simulink model "dynamic"  (R2023b)
settings: Solver=VariableStepAuto  StartTime=0.0  StopTime=5  MaxStep=1e-5  RelTol=1e-3
values from neighbouring files (symbols this model uses):
  phi0 = 0    [main.m]
  phidot0 = 0    [main.m]
  psif0 = 0    [main.m]
  psifdot0 = 0    [main.m]
  psir0 = 0    [main.m]
  psirdot0 = 0    [main.m]
  rho0 = 0    [main.m]
  rhodot0 = 0    [main.m]
  theta_dot_fl0 = xdot0*cos(car.toe.fl*pi/180)/car.tr.fl    [main.m]
  theta_dot_fr0 = xdot0*cos(car.toe.fr*pi/180)/car.tr.fr    [main.m]
  theta_dot_rl0 = xdot0*cos(car.toe.rl*pi/180)/car.tr.rl    [main.m]
  theta_dot_rr0 = xdot0*cos(car.toe.rr*pi/180)/car.tr.rr    [main.m]
  x0 = 0    [main.m]
  xdot0 = 10    [main.m]
  y0 = 0    [main.m]
  ydot0 = 0    [main.m]
  Zs0 = 0    [main.m]
  Zsdot0 = 0    [main.m]
  Zufl0 = 0    [main.m]
  Zufldot0 = 0    [main.m]
  Zufr0 = 0    [main.m]
  Zufrdot0 = 0    [main.m]
  Zurl0 = 0    [main.m]
  Zurldot0 = 0    [main.m]
  Zurr0 = 0    [main.m]
  Zurrdot0 = 0    [main.m]
undefined symbols (not defined in the file or in its folder): car
libraries: simulink x4, spsFirstOrderFilterLib x1
(part 1 of 2)
settings Model: Creator=Admin  LastModifiedBy=nathan

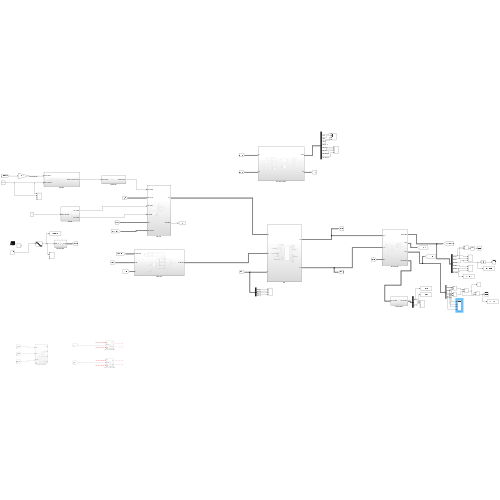
[thumbnail: Simulink's stored preview of the top-level diagram]
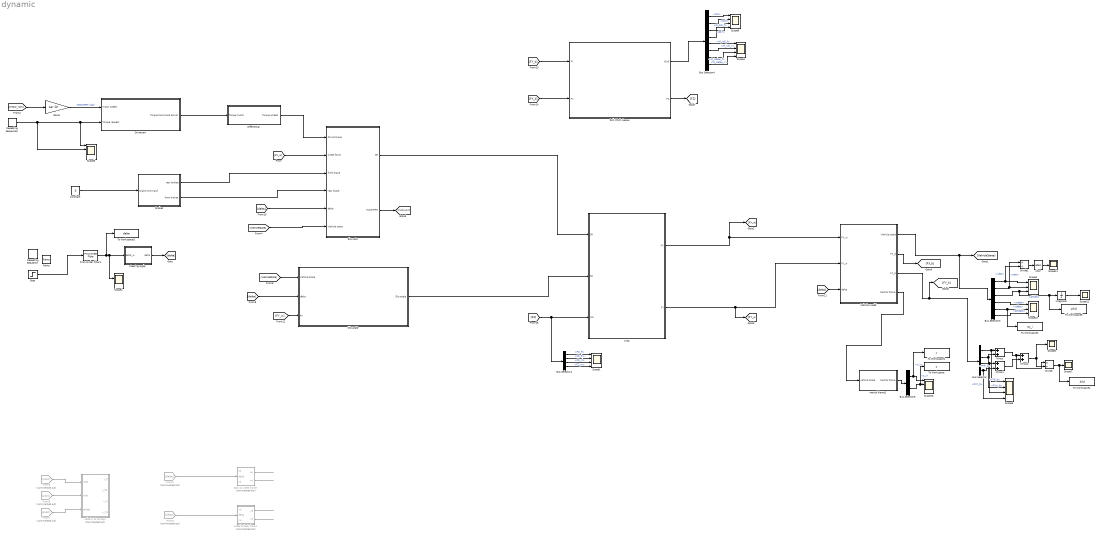
== system dynamic ==
  Atan : Trigonometry  Operator=atan
  Brakes : Subsystem
  Bus Selector : BusSelector  OutputSignals=FYfr_b,FYfl_b,FYrr_b,FYrl_b
  Bus Selector1 : BusSelector  OutputSignals=FZ_fl,FZ_fr,FZ_rl,FZ_rr
  Bus Selector3 : BusSelector  OutputSignals=xdot,ydot,phidot,xddot,yddot,phiddot
  Bus Selector4 : BusSelector  OutputSignals=cts,psif.psif,psir.psir,M_arb.M_arb_f,Roll moment.M_roll_f,Roll moment.M_roll_r,Roll moment.M_inelas_f,Roll moment.M_inelas_r
  Bus Selector5 : BusSelector  OutputSignals=x_i,y_i
  Constant : Constant  Value=0
  Differential : Subsystem
  Divide : Product  Inputs=*/
  Divide1 : Product  Inputs=*/
  Drivetrain : Subsystem
  First-Order Filter1 : spsFirstOrderFilterLib/First-Order Filter  FilterType=Lowpass  Tc=0  Ts=0  Initialize=on  Vac_Init=[0, 0, 60]  Vdc_Init=0  PlotResponse=off  FreqRange="[0,  200,  1]"
  From1 : From  Commented=on  GotoTag=delta
  From3 : From  Commented=on  GotoTag=delta
  From5 : From  Commented=on  GotoTag=xdot
  From6 : From  Commented=on  GotoTag=ydot
  From7 : From  Commented=on  GotoTag=phidot
  Gain5 : Gain  Gain=car.Gr
  Inertial frame2 : Subsystem
  Integrator : Integrator
  Minus : Sum
  Minus1 : Sum
  Minus2 : Sum
  Ramp : simulink/Sources/Ramp  slope=1  start=1  InitialOutput=0
  Repeating Sequence : simulink/Sources/Repeating Sequence  rep_seq_t=[0 1 1.1 10]  rep_seq_y=[0 0 10 25]
  Repeating Sequence2 : simulink/Sources/Repeating Sequence  rep_seq_t=[0 0.05 1 1.05 2 2.05 20]  rep_seq_y=[0 0 0 0 0 0 0]
  "Roll, Pitch, Heave" : Subsystem
  Scope{1,3..6,9,13} (7 alike) : Scope  NumInputPorts=4
  Scope10 : Scope  NumInputPorts=3
  Scope{7..8,11..12} (4 alike) : Scope
  Scope2 : Scope  NumInputPorts=3
  Slip angle : Subsystem
  Slip ratio : Subsystem
  Step : Step  After=10  SampleTime=0
  To Workspace : ToWorkspace  VariableName=y  SampleTime=-1
  To Workspace1 : ToWorkspace  VariableName=x  SampleTime=-1
  To Workspace2 : ToWorkspace  VariableName=ay_i  SampleTime=-1
  To Workspace3 : ToWorkspace  VariableName=delta  SampleTime=-1
  To Workspace4 : ToWorkspace  VariableName=AYd  SaveFormat=Timeseries  SampleTime=-1
  To Workspace5 : ToWorkspace  VariableName=phid  SaveFormat=Timeseries  SampleTime=-1
  Vehicle model : Subsystem
  body to wheel frame : Subsystem  Commented=on
  steering angle : Subsystem
  tires : Subsystem
  velocity at corners : Subsystem  Commented=on
  wheel to body frame : Subsystem  Commented=on
  wires:
  [motor_rpm] -> Gain5/1
  Gain5/1 -> Drivetrain/1(motor speed)  "MotorRPM (rad)"
  Constant/1 -> Brakes/1(brake command)
  ? -> body to wheel frame/1(xb)
  From1/1 -> body to wheel frame/2(delta)
  ? -> body to wheel frame/3(yb)
  body to wheel frame/1(xw) -> ?
  body to wheel frame/2(yw) -> ?
  wheel to body frame/2(yb) -> ?
  wheel to body frame/1(xb) -> ?
  ? -> wheel to body frame/3(yw)
  From3/1 -> wheel to body frame/2(delta)
  ? -> wheel to body frame/1(xw)
  From5/1 -> velocity at corners/1(xdot)
  From6/1 -> velocity at corners/2(ydot)
  From7/1 -> velocity at corners/3(phidot)
  [FX_w] -> Slip ratio/2(wheel force)
  Brakes/1(rear brakes) -> Slip ratio/3(front brake)
  Brakes/2(front brakes) -> Slip ratio/4(rear brake)
  steering angle/1(delta) -> [delta]
  [delta] -> Slip ratio/5(delta)
  [delta] -> Vehicle model/3(delta)
  Vehicle model/1(Vehicle state) -> Bus Selector3/1, [VehicleState]
  [VehicleState] -> Slip ratio/6(Vehicle state)
  [VehicleState] -> Slip angle/1(Vehicle state)
  [delta] -> Slip angle/2(delta)
  [FY_w] -> Slip angle/3(FY)
  Vehicle model/4(Inertial frame) -> Inertial frame2/1(vehicle state)
  Slip ratio/2(MotorRPM) -> [motor_rpm]
  Drivetrain/1(Torque Command actual) -> Differential/1(Torque motor)
  Differential/1(Torque wheels) -> Slip ratio/1(Drive torque)
  [FX_b] -> "Roll, Pitch, Heave"/2(FX)
  Vehicle model/2(FX_b) -> [FX_b]
  Vehicle model/3(FY_b) -> Bus Selector/1, [FY_b]
  "Roll, Pitch, Heave"/1(BUS) -> Bus Selector4/1
  "Roll, Pitch, Heave"/2(FZ) -> [FZ]
  tires/2(FY) -> Vehicle model/2(FY_w), [FY_w]
  tires/1(FX) -> [FX_w], Vehicle model/1(FX_w)
  Slip ratio/1(SR) -> tires/1(SR)
  Slip angle/1(Slip angle) -> tires/2(SA)
  [FZ] -> Bus Selector1/1, tires/3(In3)
  Bus Selector1/1 -> Scope1/1  "<FZ_fl>"
  Bus Selector1/2 -> Scope1/2  "<FZ_fr>"
  Bus Selector1/3 -> Scope1/3  "<FZ_rl>"
  Bus Selector1/4 -> Scope1/4  "<FZ_rr>"
  Bus Selector4/5 -> Scope3/1  "<M_roll_f>"
  Bus Selector4/6 -> Scope3/2  "<M_roll_r>"
  Bus Selector4/7 -> Scope3/3  "<M_inelas_f>"
  Bus Selector4/8 -> Scope3/4  "<M_inelas_r>"
  Bus Selector4/1 -> Scope6/1  "<cts>"
  Bus Selector4/2 -> Scope6/2  "<psif>"
  Bus Selector4/3 -> Scope6/3  "<psir>"
  Bus Selector4/4 -> Scope6/4  "<M_arb_f>"
  [FY_b] -> "Roll, Pitch, Heave"/1(FY)
  Repeating Sequence2/1 -> Scope5/1, Drivetrain/2(Torque request), Scope5/2
  Bus Selector3/1 -> Divide1/2, Scope2/1  "<xdot>"
  Bus Selector3/2 -> Divide1/1, Scope2/2  "<ydot>"
  Bus Selector3/3 -> To Workspace5/1, Integrator/1, Scope2/3  "<phidot>"
  Bus Selector/1 -> Scope9/1, Minus/1  "<FYfr_b>"
  Bus Selector/2 -> Minus/2, Scope9/2  "<FYfl_b>"
  Bus Selector/3 -> Scope9/3, Minus1/1  "<FYrr_b>"
  Bus Selector/4 -> Scope9/4, Minus1/2  "<FYrl_b>"
  Minus/1 -> Divide/1, Minus2/1
  Minus1/1 -> Minus2/2
  Divide/1 -> To Workspace4/1, Scope7/1
  Minus2/1 -> Scope8/1, Divide/2
  First-Order Filter1/1 -> To Workspace3/1, Scope4/2, steering angle/1(delta_w)
  Bus Selector3/4 -> Scope10/1  "<xddot>"
  Bus Selector3/5 -> Scope10/2, To Workspace2/1  "<yddot>"
  Bus Selector3/6 -> Scope10/3  "<phiddot>"
  Divide1/1 -> Atan/1
  Atan/1 -> Scope11/1
  Integrator/1 -> Scope12/1
  Inertial frame2/1(inertial frame) -> Bus Selector5/1
  Bus Selector5/1 -> To Workspace1/1, Scope13/1  "<x_i>"
  Bus Selector5/2 -> To Workspace/1, Scope13/2  "<y_i>"
  Step/1 -> First-Order Filter1/1

== system dynamic/Brakes ==
  brake command : Inport
  Gain12 : Gain  Gain=9.81*car.m
  Gain13 : Gain  Gain=car.brakebias
  Gain14 : Gain  Gain=0.5*car.tr.fr
  Gain9 : Gain  Gain=0.5*car.tr.rr
  Minus4 : Sum  Inputs=+-
  rear brakes : Outport
  front brakes : Outport  Port=2
  wires:
  Gain9/1 -> front brakes/1  "front brake"
  brake command/1 -> Gain12/1
  Gain13/1 -> Gain9/1, Minus4/2
  Gain12/1 -> Minus4/1, Gain13/1
  Minus4/1 -> Gain14/1  "rear brake torque total"
  Gain14/1 -> rear brakes/1  "rear brake"

== system dynamic/Differential ==
  Torque motor : Inport
  Gain : Gain  Gain=0.5
  Torque wheels : Outport
  wires:
  Torque motor/1 -> Gain/1
  Gain/1 -> Torque wheels/1

== system dynamic/Drivetrain ==
  motor speed : Inport
  Torque request : Inport  Port=2
  1-D Lookup Table : Lookup_n-D  NumberOfTableDimensions=1  BreakpointsForDimension1=car.motor(1,:)  Table=car.motor(2,:)  InternalRulePriority=Speed  RndMeth=Simplest
  Constant : Constant  Value=0
  Constant3 : Constant  Value=0
  Gain6 : Gain  Gain=30/pi
  Product : Product
  Saturation Dynamic : simulink/Discontinuities/Saturation Dynamic  OutMin=[]  OutMax=[]  OutDataTypeStr=Inherit: Same as second input  OutDataType=fixdt(1, 16)  OutScaling=2^-10  DoSatur=off
  Scope1 : Scope
  Scope2 : Scope
  Scope5 : Scope
  Switch : Switch  Criteria=u2 > Threshold  Threshold=7000  SaturateOnIntegerOverflow=off  InputSameDT=off
  gear ratio : Gain  Gain=car.Gr
  Torque Command actual : Outport
  wires:
  Constant3/1 -> Switch/1
  1-D Lookup Table/1 -> Saturation Dynamic/1
  Gain6/1 -> Scope2/1, Switch/2, 1-D Lookup Table/1  "MotorRPM (RPM)"
  motor speed/1 -> Product/1, Gain6/1, Product/2  "MotorRPM (rad)"
  Saturation Dynamic/1 -> Switch/3  "Torque command"
  Switch/1 -> Scope1/1, gear ratio/1  "Torque Command actual"
  Product/1 -> Scope5/1
  Constant/1 -> Saturation Dynamic/3
  Torque request/1 -> Saturation Dynamic/2
  gear ratio/1 -> Torque Command actual/1

== system dynamic/Inertial frame2 ==
  vehicle state : Inport
  Bus Creator2 : BusCreator  Inputs=3
  Bus Selector2 : BusSelector  OutputSignals=xdddot_if,yddot_if,phi
  Cos : Trigonometry  Operator=cos
  Cos1 : Trigonometry
  Integrator1 : Integrator  InitialCondition=ydot0
  Integrator2 : Integrator  InitialCondition=xdot0
  Integrator3 : Integrator  InitialCondition=x0
  Integrator4 : Integrator  InitialCondition=y0
  Minus : Sum  Inputs=+-
  Minus1 : Sum
  Product{,1..3} (4 alike) : Product
  inertial frame : Outport
  wires:
  Integrator1/1 -> Integrator4/1  "ydot_i"
  Bus Selector2/3 -> Cos/1, Bus Creator2/3, Cos1/1  "<phi>"
  Cos1/1 -> Product1/2, Product2/2
  Bus Creator2/1 -> inertial frame/1
  Bus Selector2/2 -> Product3/1, Product1/1  "<yddot_if>"
  Cos/1 -> Product/2, Product3/2
  Product3/1 -> Minus1/2
  Product2/1 -> Minus1/1
  Bus Selector2/1 -> Product2/1, Product/1  "<xdddot_if>"
  Integrator2/1 -> Integrator3/1  "xdot_i"
  Minus1/1 -> Integrator1/1  "yydot_i"
  Minus/1 -> Integrator2/1  "xdot_i"
  Product/1 -> Minus/1
  Product1/1 -> Minus/2
  vehicle state/1 -> Bus Selector2/1
  Integrator3/1 -> Bus Creator2/1  "x_i"
  Integrator4/1 -> Bus Creator2/2  "y_i"

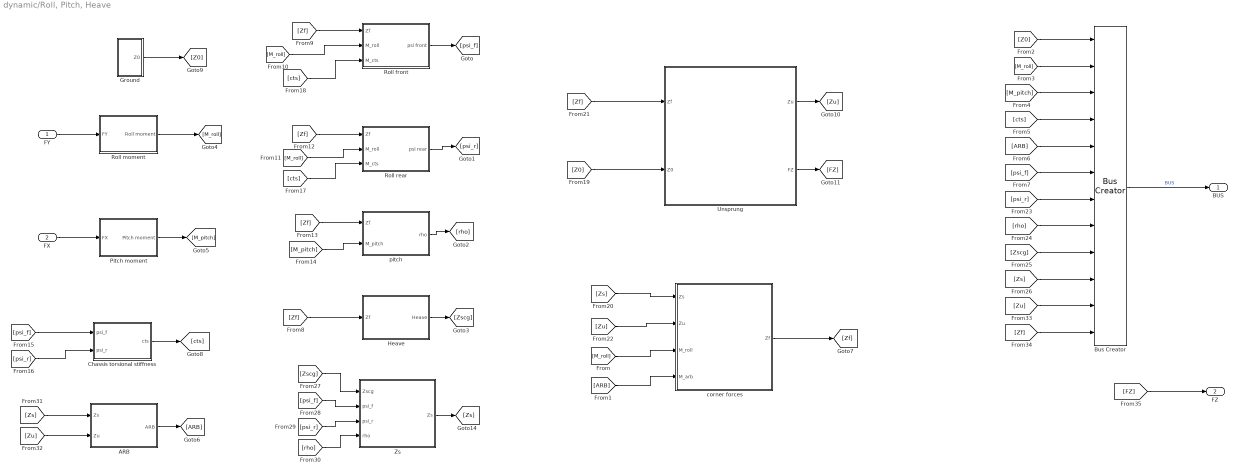
== system dynamic/Roll, Pitch, Heave ==
  FY : Inport
  FX : Inport  Port=2
  ARB : Subsystem
  Bus Creator : BusCreator  Inputs=12
  Chassis torsional stiffness : Subsystem
  Ground : Subsystem
  Heave : Subsystem
  Pitch moment : Subsystem
  Roll front : Subsystem
  Roll moment : Subsystem
  Roll rear : Subsystem
  Unsprung : Subsystem
  Zs : Subsystem
  corner forces : Subsystem
  pitch : Subsystem
  BUS : Outport
  FZ : Outport  Port=2
  wires:
  FY/1 -> Roll moment/1(FY)
  FX/1 -> Pitch moment/1(FX)
  Roll front/1(psi front) -> [psi_f]
  Roll rear/1(psi rear) -> [psi_r]
  pitch/1(rho) -> [rho]
  Heave/1(Heave) -> [Zscg]
  Roll moment/1(Roll moment) -> [M_roll]
  Pitch moment/1(Pitch moment) -> [M_pitch]
  ARB/1(ARB) -> [ARB]
  [Zf] -> Heave/1(Zf)
  [Zf] -> Roll front/1(Zf)
  [M_roll] -> Roll front/2(M_roll)
  [M_roll] -> Roll rear/2(M_roll)
  [Zf] -> Roll rear/1(Zf)
  [Zf] -> pitch/1(Zf)
  [M_pitch] -> pitch/2(M_pitch)
  Chassis torsional stiffness/1(cts) -> [cts]
  [psi_f] -> Chassis torsional stiffness/1(psi_f)
  [psi_r] -> Chassis torsional stiffness/2(psi_r)
  [cts] -> Roll front/3(M_cts)
  [cts] -> Roll rear/3(M_cts)
  Ground/1(Z0) -> [Z0]
  [Zscg] -> Zs/1(Zscg)
  [psi_f] -> Zs/2(psi_f)
  [psi_r] -> Zs/3(psi_r)
  [rho] -> Zs/4(rho)
  Zs/1(Zs) -> [Zs]
  [Zs] -> ARB/1(Zs)
  [Zf] -> Unsprung/1(Zf)
  [Z0] -> Unsprung/2(Z0)
  Unsprung/1(Zu) -> [Zu]
  [Zu] -> ARB/2(Zu)
  [Zs] -> corner forces/1(Zs)
  [Zu] -> corner forces/2(Zu)
  [M_roll] -> corner forces/3(M_roll)
  [ARB] -> corner forces/4(M_arb)
  corner forces/1(Zf) -> [Zf]
  [Z0] -> Bus Creator/1
  [M_roll] -> Bus Creator/2
  [M_pitch] -> Bus Creator/3
  [cts] -> Bus Creator/4
  [ARB] -> Bus Creator/5
  [psi_f] -> Bus Creator/6
  [psi_r] -> Bus Creator/7
  [rho] -> Bus Creator/8
  [Zscg] -> Bus Creator/9
  [Zs] -> Bus Creator/10
  [Zu] -> Bus Creator/11
  [Zf] -> Bus Creator/12
  Bus Creator/1 -> BUS/1  "BUS"
  Unsprung/2(FZ) -> [FZ]
  [FZ] -> FZ/1

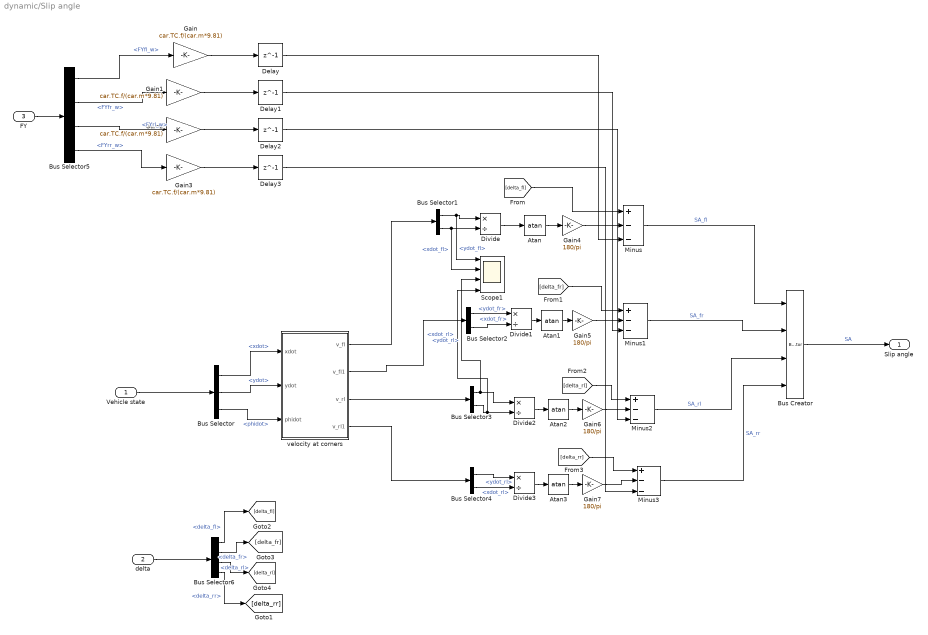
== system dynamic/Slip angle ==
  Vehicle state : Inport
  delta : Inport  Port=2
  FY : Inport  Port=3
  Atan{,1..3} (4 alike) : Trigonometry  Operator=atan
  Bus Creator : BusCreator  Inputs=4
  Bus Selector : BusSelector  OutputSignals=xdot,ydot,phidot
  Bus Selector1 : BusSelector  OutputSignals=ydot_fl,xdot_fl
  Bus Selector2 : BusSelector  OutputSignals=ydot_fr,xdot_fr
  Bus Selector3 : BusSelector  OutputSignals=ydot_rl,xdot_rl
  Bus Selector4 : BusSelector  OutputSignals=ydot_rl,xdot_rl
  Bus Selector5 : BusSelector  OutputSignals=FYfl_w,FYfr_w,FYrl_w,FYrr_w
  Bus Selector6 : BusSelector  OutputSignals=delta_fl,delta_fr,delta_rl,delta_rr
  Delay{,1..3} (4 alike) : Delay  DelayLength=1
  Divide{,1..3} (4 alike) : Product  Inputs=*/
  Gain{,1..3} (4 alike) : Gain  Gain=car.TC.f/(car.m*9.81)
  Gain{4..7} (4 alike) : Gain  Gain=180/pi
  Minus{,1..3} (4 alike) : Sum  Inputs=+--
  Scope1 : Scope  NumInputPorts=4
  velocity at corners : Subsystem
  Slip angle : Outport
  wires:
  Vehicle state/1 -> Bus Selector/1
  Bus Selector/1 -> velocity at corners/1(xdot)  "<xdot>"
  Bus Selector/2 -> velocity at corners/2(ydot)  "<ydot>"
  Bus Selector/3 -> velocity at corners/3(phidot)  "<phidot>"
  velocity at corners/1(v_fl) -> Bus Selector1/1
  Bus Selector1/1 -> Scope1/1, Divide/1  "<ydot_fl>"
  Bus Selector1/2 -> Scope1/2, Divide/2  "<xdot_fl>"
  Divide/1 -> Atan/1
  Divide1/1 -> Atan1/1
  velocity at corners/2(v_fl1) -> Bus Selector2/1
  Divide2/1 -> Atan2/1
  Divide3/1 -> Atan3/1
  velocity at corners/3(v_rl) -> Bus Selector3/1
  velocity at corners/4(v_rl1) -> Bus Selector4/1
  Bus Selector4/1 -> Divide3/1  "<ydot_rl>"
  Bus Selector4/2 -> Divide3/2  "<xdot_rl>"
  Bus Selector3/1 -> Scope1/3, Divide2/1  "<ydot_rl>"
  Bus Selector3/2 -> Divide2/2, Scope1/4  "<xdot_rl>"
  Bus Selector2/1 -> Divide1/1  "<ydot_fr>"
  Bus Selector2/2 -> Divide1/2  "<xdot_fr>"
  Atan/1 -> Gain4/1
  Bus Selector6/2 -> [delta_fr]  "<delta_fr>"
  Bus Selector6/4 -> [delta_rr]  "<delta_rr>"
  Bus Selector6/3 -> [delta_rl]  "<delta_rl>"
  Bus Selector6/1 -> [delta_fl]  "<delta_fl>"
  delta/1 -> Bus Selector6/1
  [delta_fl] -> Minus/1
  Atan1/1 -> Gain5/1
  [delta_fr] -> Minus1/1
  Atan3/1 -> Gain7/1
  Atan2/1 -> Gain6/1
  [delta_rl] -> Minus2/1
  [delta_rr] -> Minus3/1
  FY/1 -> Bus Selector5/1
  Bus Selector5/1 -> Gain/1  "<FYfl_w>"
  Bus Selector5/2 -> Gain1/1  "<FYfr_w>"
  Bus Selector5/3 -> Gain2/1  "<FYrl_w>"
  Bus Selector5/4 -> Gain3/1  "<FYrr_w>"
  Gain/1 -> Delay/1
  Gain1/1 -> Delay1/1
  Gain2/1 -> Delay2/1
  Gain3/1 -> Delay3/1
  Minus/1 -> Bus Creator/1  "SA_fl"
  Minus1/1 -> Bus Creator/2  "SA_fr"
  Minus2/1 -> Bus Creator/3  "SA_rl"
  Minus3/1 -> Bus Creator/4  "SA_rr"
  Bus Creator/1 -> Slip angle/1  "SA"
  Delay/1 -> Minus/3
  Delay1/1 -> Minus1/3
  Delay2/1 -> Minus2/3
  Delay3/1 -> Minus3/3
  Gain4/1 -> Minus/2
  Gain5/1 -> Minus1/2
  Gain6/1 -> Minus2/2
  Gain7/1 -> Minus3/2

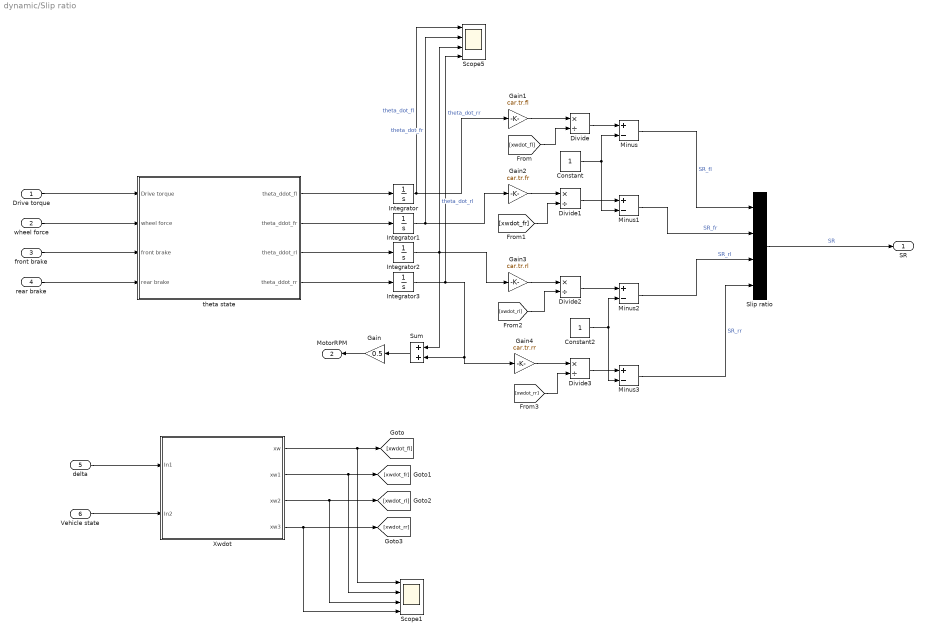
== system dynamic/Slip ratio ==
  Drive torque : Inport
  wheel force : Inport  Port=2
  front brake : Inport  Port=3
  rear brake : Inport  Port=4
  delta : Inport  Port=5
  Vehicle state : Inport  Port=6
  Constant : Constant
  Constant2 : Constant
  Divide{,1..3} (4 alike) : Product  Inputs=*/
  Gain : Gain  Gain=0.5
  Gain1 : Gain  Gain=car.tr.fl
  Gain2 : Gain  Gain=car.tr.fr
  Gain3 : Gain  Gain=car.tr.rl
  Gain4 : Gain  Gain=car.tr.rr
  Integrator : Integrator  InitialCondition=theta_dot_fr0
  Integrator1 : Integrator  InitialCondition=theta_dot_fl0
  Integrator2 : Integrator  InitialCondition=theta_dot_rl0
  Integrator3 : Integrator  InitialCondition=theta_dot_rr0
  Minus{,1..3} (4 alike) : Sum  Inputs=+-
  Scope1 : Scope  NumInputPorts=4
  Scope5 : Scope  NumInputPorts=4
  Slip ratio : BusCreator  Inputs=4
  Sum : Sum
  Xwdot : Subsystem
  theta state : Subsystem
  SR : Outport
  MotorRPM : Outport  Port=2
  wires:
  Integrator3/1 -> Scope5/4, Sum/2, Gain4/1  "theta_dot_rr"
  Integrator/1 -> Scope5/1, Gain1/1  "theta_dot_fl"
  Integrator2/1 -> Scope5/3, Sum/1, Gain3/1  "theta_dot_rl"
  theta state/3(theta_ddot_rl) -> Integrator2/1
  theta state/4(theta_ddot_rr) -> Integrator3/1
  theta state/2(theta_ddot_fr) -> Integrator1/1
  Integrator1/1 -> Scope5/2, Gain2/1  "theta_dot_fr"
  theta state/1(theta_ddot_fl) -> Integrator/1
  wheel force/1 -> theta state/2(wheel force)
  Gain2/1 -> Divide1/1
  Drive torque/1 -> theta state/1(Drive torque)
  Gain3/1 -> Divide2/1
  front brake/1 -> theta state/3(front brake)
  rear brake/1 -> theta state/4(rear brake)
  Gain1/1 -> Divide/1
  [xwdot_fl] -> Divide/2
  [xwdot_fr] -> Divide1/2
  [xwdot_rl] -> Divide2/2
  [xwdot_rr] -> Divide3/2
  Gain4/1 -> Divide3/1
  Divide/1 -> Minus/1
  Constant/1 -> Minus/2, Minus1/2
  Divide1/1 -> Minus1/1
  Divide2/1 -> Minus2/1
  Divide3/1 -> Minus3/1
  Constant2/1 -> Minus2/2, Minus3/2
  Minus/1 -> Slip ratio/1  "SR_fl"
  Minus1/1 -> Slip ratio/2  "SR_fr"
  Minus2/1 -> Slip ratio/3  "SR_rl"
  Minus3/1 -> Slip ratio/4  "SR_rr"
  Slip ratio/1 -> SR/1  "SR"
  delta/1 -> Xwdot/1(In1)
  Vehicle state/1 -> Xwdot/2(In2)
  Xwdot/2(xw1) -> Scope1/2, [xwdot_fr]
  Xwdot/3(xw2) -> Scope1/3, [xwdot_rl]
  Xwdot/4(xw3) -> Scope1/4, [xwdot_rr]
  Sum/1 -> Gain/1
  Gain/1 -> MotorRPM/1
  Xwdot/1(xw) -> Scope1/1, [xwdot_fl]

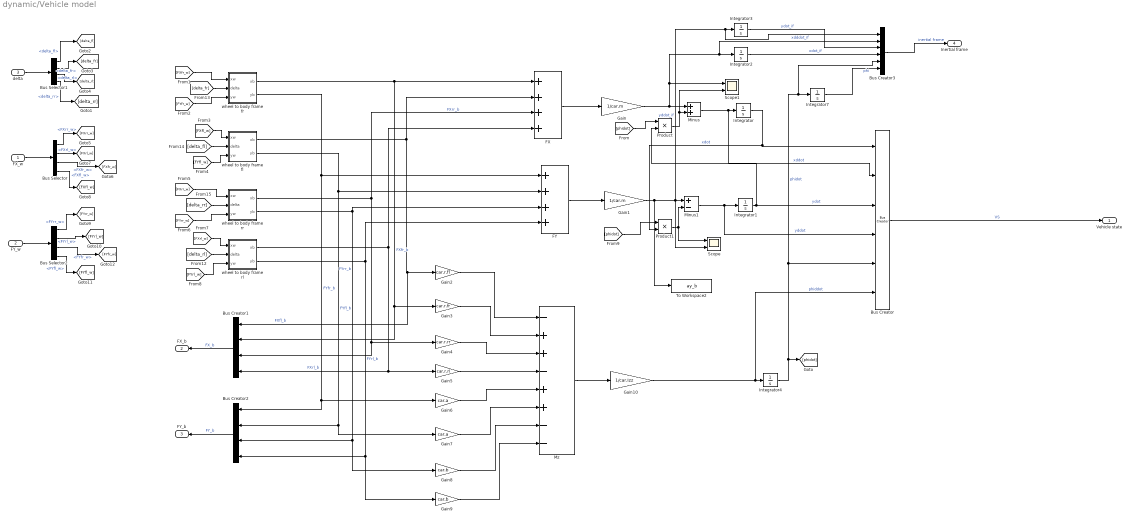
== system dynamic/Vehicle model ==
  FX_w : Inport
  FY_w : Inport  Port=2
  delta : Inport  Port=3
  Bus Creator : BusCreator  Inputs=6
  Bus Creator1 : BusCreator  Inputs=4
  Bus Creator2 : BusCreator  Inputs=4
  Bus Creator3 : BusCreator  Inputs=6
  Bus Selector : BusSelector  OutputSignals=FXrr_w,FXrl_w,FXfr_w,FXfl_w
  Bus Selector1 : BusSelector  OutputSignals=delta_fl,delta_fr,delta_rl,delta_rr
  Bus Selector2 : BusSelector  OutputSignals=FYrr_w,FYrl_w,FYfr_w,FYfl_w
  FX : Sum  Inputs=++++
  FY : Sum  Inputs=++++
  Gain : Gain  Gain=1/car.m
  Gain1 : Gain  Gain=1/car.m
  Gain10 : Gain  Gain=1/car.Izz
  Gain2 : Gain  Gain=car.r.fl
  Gain3 : Gain  Gain=car.r.fr
  Gain4 : Gain  Gain=car.r.rr
  Gain5 : Gain  Gain=car.r.rl
  Gain6 : Gain  Gain=car.a
  Gain7 : Gain  Gain=car.a
  Gain8 : Gain  Gain=car.b
  Gain9 : Gain  Gain=car.b
  Integrator : Integrator  InitialCondition=xdot0
  Integrator1 : Integrator  InitialCondition=ydot0
  Integrator2 : Integrator  InitialCondition=xdot0
  Integrator3 : Integrator
  Integrator4 : Integrator  InitialCondition=phidot0
  Integrator7 : Integrator  InitialCondition=phi0
  Minus : Sum
  Minus1 : Sum  Inputs=+-
  Mz : Sum  Inputs=-++-++--
  Product : Product
  Product1 : Product
  Scope : Scope  NumInputPorts=2
  Scope1 : Scope  NumInputPorts=2
  To Workspace2 : ToWorkspace  VariableName=ay_b  SampleTime=-1
  wheel to body frame fl : Subsystem
  wheel to body frame fr : Subsystem
  wheel to body frame rl : Subsystem
  wheel to body frame rr : Subsystem
  Vehicle state : Outport
  FX_b : Outport  Port=2
  FY_b : Outport  Port=3
  Inertial frame : Outport  Port=4
  wires:
  [delta_fl] -> wheel to body frame fl/2(delta)
  delta/1 -> Bus Selector1/1
  Bus Selector1/3 -> [delta_rl]  "<delta_rl>"
  [delta_fr] -> wheel to body frame fr/2(delta)
  [delta_rr] -> wheel to body frame rr/2(delta)
  Bus Selector1/2 -> [delta_fr]  "<delta_fr>"
  Bus Selector1/1 -> [delta_fl]  "<delta_fl>"
  Bus Selector1/4 -> [delta_rr]  "<delta_rr>"
  [delta_rl] -> wheel to body frame rl/2(delta)
  wheel to body frame rr/2(yb) -> FY/3, Bus Creator2/3, Gain8/1  "FYrr_b"
  wheel to body frame fr/1(xb) -> Bus Creator1/2, Gain3/1, FX/1  "FXfr_b"
  wheel to body frame fl/2(yb) -> Bus Creator2/2, Gain7/1, FY/2  "FYfl_b"
  wheel to body frame rl/1(xb) -> FX/4, Bus Creator1/4, Gain5/1  "FXrl_b"
  wheel to body frame rl/2(yb) -> FY/4, Bus Creator2/4, Gain9/1  "FYrl_b"
  wheel to body frame fl/1(xb) -> FX/2, Bus Creator1/1, Gain2/1  "FXfl_b"
  FX_w/1 -> Bus Selector/1
  FY_w/1 -> Bus Selector2/1
  Bus Selector/1 -> [FXrr_w]  "<FXrr_w>"
  Bus Selector/2 -> [FXrl_w]  "<FXrl_w>"
  Bus Selector/3 -> [FXfr_w]  "<FXfr_w>"
  Bus Selector/4 -> [FXfl_w]  "<FXfl_w>"
  Bus Selector2/1 -> [FYrr_w]  "<FYrr_w>"
  Bus Selector2/2 -> [FYrl_w]  "<FYrl_w>"
  Bus Selector2/3 -> [FYfr_w]  "<FYfr_w>"
  Bus Selector2/4 -> [FYfl_w]  "<FYfl_w>"
  [FXfr_w] -> wheel to body frame fr/1(xw)
  [FYfr_w] -> wheel to body frame fr/3(yw)
  [FXfl_w] -> wheel to body frame fl/1(xw)
  [FYfl_w] -> wheel to body frame fl/3(yw)
  [FXrr_w] -> wheel to body frame rr/1(xw)
  [FYrr_w] -> wheel to body frame rr/3(yw)
  [FXrl_w] -> wheel to body frame rl/1(xw)
  [FYrl_w] -> wheel to body frame rl/3(yw)
  wheel to body frame rr/1(xb) -> FX/3, Bus Creator1/3, Gain4/1  "FXrr_b"
  wheel to body frame fr/2(yb) -> Bus Creator2/1, Gain6/1, FY/1  "FYfr_b"
  FX/1 -> Gain/1
  FY/1 -> Gain1/1
  Integrator1/1 -> Product/2, Bus Creator/3  "ydot"
  Integrator/1 -> Bus Creator/1, Product1/2  "xdot"
  Gain2/1 -> Mz/1
  Gain3/1 -> Mz/2
  Gain4/1 -> Mz/3
  Gain5/1 -> Mz/4
  Gain6/1 -> Mz/5
  Gain7/1 -> Mz/6
  Gain8/1 -> Mz/7
  Gain9/1 -> Mz/8
  Mz/1 -> Gain10/1
  Gain10/1 -> Bus Creator/6, Integrator4/1  "phiddot"
  Integrator4/1 -> Bus Creator3/5, Integrator7/1, Bus Creator/5, [phidot]  "phidot"
  Gain/1 -> Bus Creator3/2, Integrator2/1, Scope1/1, Minus/1  "xdddot_if"
  Minus1/1 -> Bus Creator/4, Integrator1/1  "yddot"
  [phidot] -> Product/1
  [phidot] -> Product1/1
  Bus Creator/1 -> Vehicle state/1  "VS"
  Bus Creator1/1 -> FX_b/1  "FX_b"
  Bus Creator2/1 -> FY_b/1  "FY_b"
  Gain1/1 -> To Workspace2/1, Bus Creator3/1, Integrator3/1, Scope/2, Minus1/1  "yddot_if"
  Minus/1 -> Bus Creator/2, Integrator/1  "xddot"
  Product/1 -> Scope1/2, Minus/2
  Product1/1 -> Minus1/2, Scope/1
  Bus Creator3/1 -> Inertial frame/1  "inertial frame"
  Integrator7/1 -> Bus Creator3/6  "phi"
  Integrator3/1 -> Bus Creator3/3  "ydot_if"
  Integrator2/1 -> Bus Creator3/4  "xdot_if"

== system dynamic/body to wheel frame ==
  xb : Inport
  delta : Inport  Port=2
  yb : Inport  Port=3
  Cos : Trigonometry  Operator=cos
  Cos1 : Trigonometry
  Minus : Sum
  Minus1 : Sum  Inputs=-+
  Product{,1..3} (4 alike) : Product
  xw : Outport
  yw : Outport  Port=2
  wires:
  Cos/1 -> Product3/2, Product/2
  Product2/1 -> Minus1/1
  Cos1/1 -> Product2/2, Product1/1
  yb/1 -> Product3/1, Product1/2
  Product1/1 -> Minus/2
  delta/1 -> Cos1/1, Cos/1
  Minus/1 -> xw/1
  Product3/1 -> Minus1/2
  Product/1 -> Minus/1
  xb/1 -> Product2/1, Product/1
  Minus1/1 -> yw/1

== system dynamic/steering angle ==
  delta_w : Inport
  Bus Creator : BusCreator  Inputs=4
  Constant : Constant  Value=0
  Constant1 : Constant  Value=car.toe.fl
  Constant2 : Constant  Value=car.toe.fr
  Constant3 : Constant  Value=car.toe.rl
  Constant4 : Constant  Value=car.toe.rr
  Minus{,1..3} (4 alike) : Sum
  Scope4 : Scope  NumInputPorts=4
  delta : Outport
  wires:
  delta_w/1 -> Minus1/1, Minus/1
  Constant1/1 -> Minus/2
  Constant4/1 -> Minus3/2
  Constant3/1 -> Minus2/2
  Minus3/1 -> Bus Creator/4, Scope4/4  "delta_rr"
  Minus/1 -> Scope4/1, Bus Creator/1  "delta_fl"
  Constant2/1 -> Minus1/2
  Minus1/1 -> Scope4/2, Bus Creator/2  "delta_fr"
  Minus2/1 -> Scope4/3, Bus Creator/3  "delta_rl"
  Bus Creator/1 -> delta/1  "delta"
  Constant/1 -> Minus3/1, Minus2/1

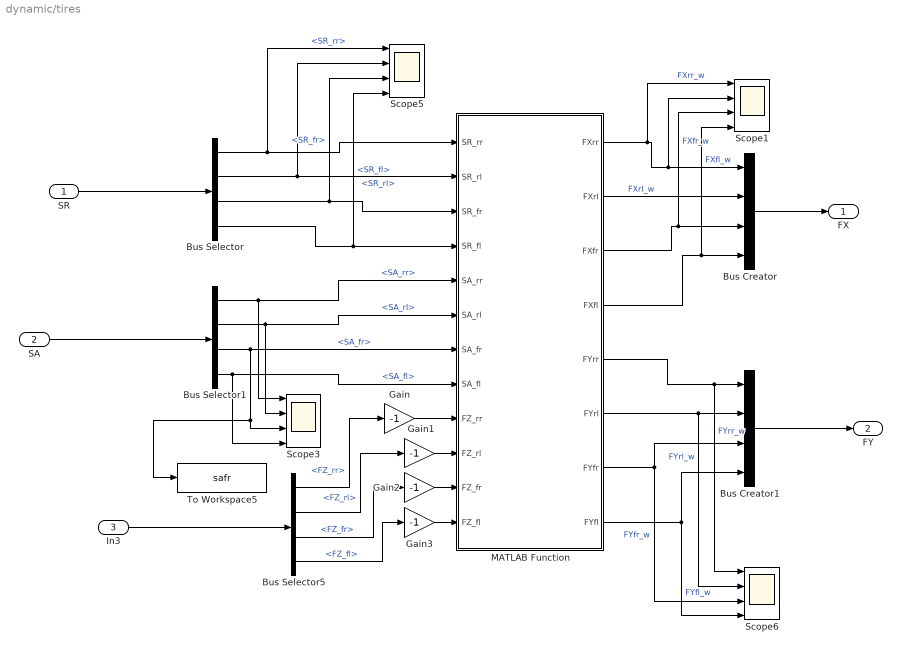
== system dynamic/tires ==
  SR : Inport
  SA : Inport  Port=2
  In3 : Inport  Port=3
  Bus Creator : BusCreator  Inputs=4
  Bus Creator1 : BusCreator  Inputs=4
  Bus Selector : BusSelector  OutputSignals=SR_rr,SR_rl,SR_fr,SR_fl
  Bus Selector1 : BusSelector  OutputSignals=SA_rr,SA_rl,SA_fr,SA_fl
  Bus Selector5 : BusSelector  OutputSignals=FZ_rr,FZ_rl,FZ_fr,FZ_fl
  Gain{,1..3} (4 alike) : Gain  Gain=-1
  MATLAB Function : MATLAB Function  TreatAsAtomicUnit=on
  Scope{1,3,5..6} (4 alike) : Scope  NumInputPorts=4
  To Workspace5 : ToWorkspace  VariableName=safr  SaveFormat=Timeseries  SampleTime=-1
  FX : Outport
  FY : Outport  Port=2
  wires:
  MATLAB Function/1(FXrr) -> Scope1/1, Scope1/2, Bus Creator/1  "FXrr_w"
  Bus Selector1/1 -> MATLAB Function/5(SA_rr), Scope3/1  "<SA_rr>"
  Bus Selector/4 -> Scope5/4, MATLAB Function/4(SR_fl)  "<SR_fl>"
  MATLAB Function/2(FXrl) -> Bus Creator/2  "FXrl_w"
  Bus Selector/2 -> Scope5/2, MATLAB Function/2(SR_rl)  "<SR_rl>"
  Bus Selector1/2 -> Scope3/2, MATLAB Function/6(SA_rl)  "<SA_rl>"
  Bus Selector1/4 -> Scope3/4, MATLAB Function/8(SA_fl)  "<SA_fl>"
  Bus Selector/1 -> Scope5/1, MATLAB Function/1(SR_rr)  "<SR_rr>"
  MATLAB Function/5(FYrr) -> Scope6/1, Bus Creator1/1  "FYrr_w"
  MATLAB Function/3(FXfr) -> Scope1/3, Bus Creator/3  "FXfr_w"
  Bus Selector1/3 -> To Workspace5/1, Scope3/3, MATLAB Function/7(SA_fr)  "<SA_fr>"
  Bus Selector/3 -> Scope5/3, MATLAB Function/3(SR_fr)  "<SR_fr>"
  MATLAB Function/6(FYrl) -> Scope6/2, Bus Creator1/2  "FYrl_w"
  Bus Selector5/1 -> Gain/1  "<FZ_rr>"
  MATLAB Function/7(FYfr) -> Bus Creator1/3, Scope6/3  "FYfr_w"
  MATLAB Function/4(FXfl) -> Scope1/4, Bus Creator/4  "FXfl_w"
  Bus Selector5/2 -> Gain1/1  "<FZ_rl>"
  Bus Selector5/4 -> Gain3/1  "<FZ_fl>"
  SR/1 -> Bus Selector/1
  In3/1 -> Bus Selector5/1
  Bus Selector5/3 -> Gain2/1  "<FZ_fr>"
  MATLAB Function/8(FYfl) -> Bus Creator1/4, Scope6/4  "FYfl_w"
  SA/1 -> Bus Selector1/1
  Bus Creator/1 -> FX/1
  Bus Creator1/1 -> FY/1
  Gain/1 -> MATLAB Function/9(FZ_rr)
  Gain1/1 -> MATLAB Function/10(FZ_rl)
  Gain2/1 -> MATLAB Function/11(FZ_fr)
  Gain3/1 -> MATLAB Function/12(FZ_fl)

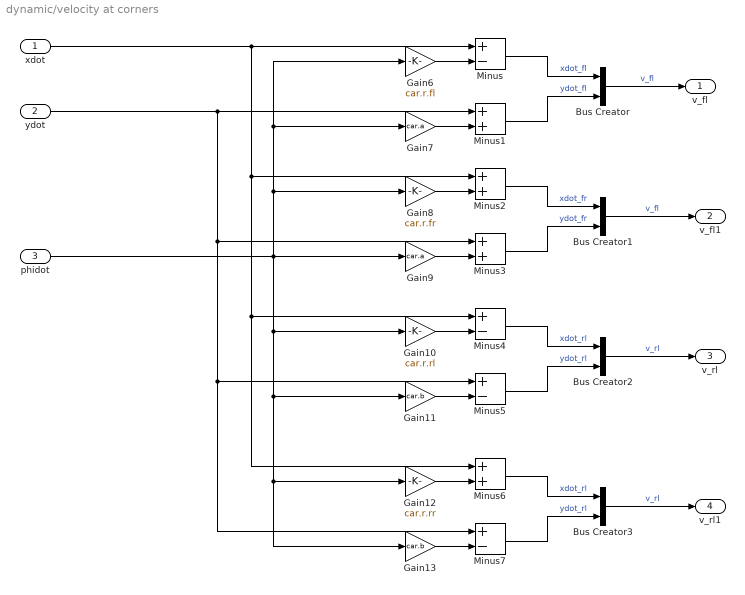
== system dynamic/velocity at corners ==
  xdot : Inport
  ydot : Inport  Port=2
  phidot : Inport  Port=3
  Bus Creator{,1..3} (4 alike) : BusCreator  Inputs=2
  Gain10 : Gain  Gain=car.r.rl
  Gain11 : Gain  Gain=car.b
  Gain12 : Gain  Gain=car.r.rr
  Gain13 : Gain  Gain=car.b
  Gain6 : Gain  Gain=car.r.fl
  Gain7 : Gain  Gain=car.a
  Gain8 : Gain  Gain=car.r.fr
  Gain9 : Gain  Gain=car.a
  Minus{,4..5,7} (4 alike) : Sum  Inputs=+-
  Minus{1..3,6} (4 alike) : Sum
  v_fl : Outport
  v_fl1 : Outport  Port=2
  v_rl : Outport  Port=3
  v_rl1 : Outport  Port=4
  wires:
  ydot/1 -> Minus7/1, Minus5/1, Minus3/1, Minus1/1
  Gain8/1 -> Minus2/2
  Gain7/1 -> Minus1/2
  phidot/1 -> Gain7/1, Gain6/1, Gain8/1, Gain13/1, Gain12/1, Gain11/1, Gain10/1, Gain9/1
  Minus2/1 -> Bus Creator1/1  "xdot_fr"
  xdot/1 -> Minus6/1, Minus4/1, Minus2/1, Minus/1
  Minus1/1 -> Bus Creator/2  "ydot_fl"
  Gain9/1 -> Minus3/2
  Gain10/1 -> Minus4/2
  Gain11/1 -> Minus5/2
  Minus5/1 -> Bus Creator2/2  "ydot_rl"
  Minus4/1 -> Bus Creator2/1  "xdot_rl"
  Gain12/1 -> Minus6/2
  Minus7/1 -> Bus Creator3/2  "ydot_rl"
  Minus6/1 -> Bus Creator3/1  "xdot_rl"
  Gain13/1 -> Minus7/2
  Minus/1 -> Bus Creator/1  "xdot_fl"
  Gain6/1 -> Minus/2
  Minus3/1 -> Bus Creator1/2  "ydot_fr"
  Bus Creator2/1 -> v_rl/1  "v_rl"
  Bus Creator3/1 -> v_rl1/1  "v_rl"
  Bus Creator1/1 -> v_fl1/1  "v_fl"
  Bus Creator/1 -> v_fl/1  "v_fl"

== system dynamic/wheel to body frame ==
  xw : Inport
  delta : Inport  Port=2
  yw : Inport  Port=3
  Cos : Trigonometry  Operator=cos
  Cos1 : Trigonometry
  Minus : Sum  Inputs=+-
  Minus1 : Sum
  Product{,1..3} (4 alike) : Product
  xb : Outport
  yb : Outport  Port=2
  wires:
  Minus1/1 -> yb/1
  xw/1 -> Product/1, Product2/1
  Product/1 -> Minus/1
  Product3/1 -> Minus1/2
  Minus/1 -> xb/1
  delta/1 -> Cos/1, Cos1/1
  Product1/1 -> Minus/2
  yw/1 -> Product1/2, Product3/1
  Cos1/1 -> Product1/1, Product2/2
  Product2/1 -> Minus1/1
  Cos/1 -> Product/2, Product3/2

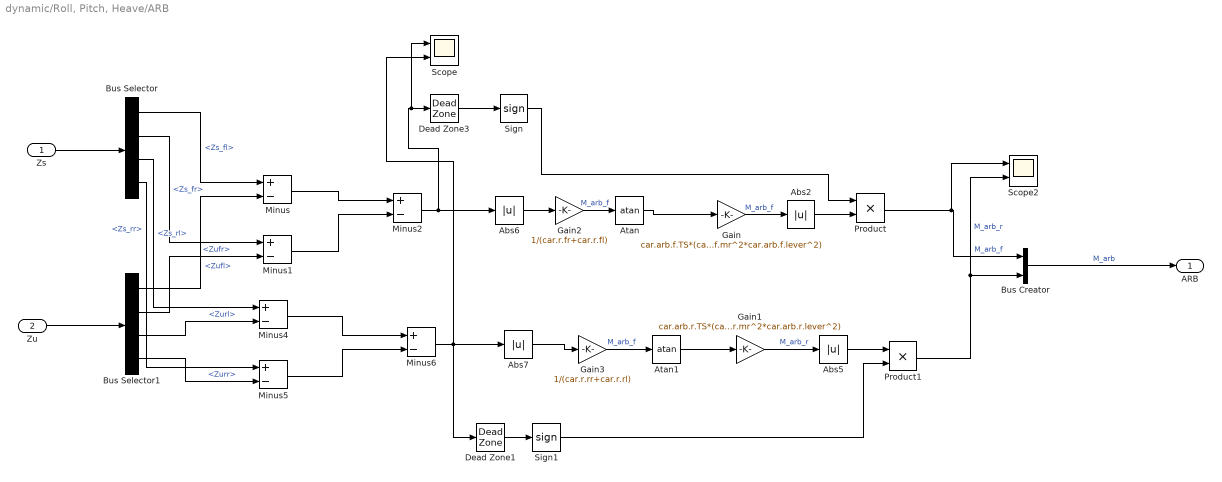
== system dynamic/Roll, Pitch, Heave/ARB ==
  Zs : Inport
  Zu : Inport  Port=2
  Abs{2,5..7} (4 alike) : Abs  ZeroCross=off  SaturateOnIntegerOverflow=off
  Atan : Trigonometry  Operator=atan
  Atan1 : Trigonometry  Operator=atan
  Bus Creator : BusCreator  Inputs=2
  Bus Selector : BusSelector  OutputSignals=Zs_fl,Zs_fr,Zs_rl,Zs_rr
  Bus Selector1 : BusSelector  OutputSignals=Zu_fl.Zufl,Zu_fr.Zufr,Zu_rl.Zurl,Zu_rr.Zurr
  Dead Zone1 : DeadZone  LowerValue=-0.0000001  UpperValue=0.0000001  ZeroCross=off
  Dead Zone3 : DeadZone  LowerValue=-0.0000001  UpperValue=0.0000001  ZeroCross=off
  Gain : Gain  Gain=car.arb.f.TS*(car.r.fr+car.r.fl)^2/(car.arb.f.mr^2*car.arb.f.lever^2)
  Gain1 : Gain  Gain=car.arb.r.TS*(car.r.rr+car.r.rl)^2/(car.arb.r.mr^2*car.arb.r.lever^2)
  Gain2 : Gain  Gain=1/(car.r.fr+car.r.fl)
  Gain3 : Gain  Gain=1/(car.r.rr+car.r.rl)
  Minus{,1..2,4..6} (6 alike) : Sum  Inputs=+-
  Product : Product
  Product1 : Product
  Scope : Scope  NumInputPorts=2
  Scope2 : Scope  NumInputPorts=2
  Sign : Signum  ZeroCross=off
  Sign1 : Signum  ZeroCross=off
  ARB : Outport
  wires:
  Bus Creator/1 -> ARB/1  "M_arb"
  Zs/1 -> Bus Selector/1
  Zu/1 -> Bus Selector1/1
  Bus Selector/1 -> Minus/1  "<Zs_fl>"
  Bus Selector1/1 -> Minus/2  "<Zufl>"
  Bus Selector/2 -> Minus1/1  "<Zs_fr>"
  Bus Selector1/2 -> Minus1/2  "<Zufr>"
  Minus/1 -> Minus2/1
  Minus1/1 -> Minus2/2
  Minus2/1 -> Scope/1, Dead Zone3/1, Abs6/1
  Sign/1 -> Product/1
  Gain/1 -> Abs2/1  "M_arb_f"
  Product/1 -> Scope2/1, Bus Creator/1  "M_arb_f"
  Abs2/1 -> Product/2
  Bus Selector/3 -> Minus4/1  "<Zs_rl>"
  Bus Selector1/3 -> Minus4/2  "<Zurl>"
  Bus Selector/4 -> Minus5/1  "<Zs_rr>"
  Bus Selector1/4 -> Minus5/2  "<Zurr>"
  Minus4/1 -> Minus6/1
  Minus5/1 -> Minus6/2
  Minus6/1 -> Dead Zone1/1, Scope/2, Abs7/1
  Gain1/1 -> Abs5/1  "M_arb_r"
  Abs5/1 -> Product1/1
  Product1/1 -> Scope2/2, Bus Creator/2  "M_arb_r"
  Sign1/1 -> Product1/2
  Dead Zone3/1 -> Sign/1
  Dead Zone1/1 -> Sign1/1
  Gain2/1 -> Atan/1  "M_arb_f"
  Atan/1 -> Gain/1
  Atan1/1 -> Gain1/1
  Gain3/1 -> Atan1/1  "M_arb_f"
  Abs6/1 -> Gain2/1
  Abs7/1 -> Gain3/1

== system dynamic/Roll, Pitch, Heave/Chassis torsional stiffness ==
  psi_f : Inport
  psi_r : Inport  Port=2
  Bus Selector : BusSelector  OutputSignals=psif
  Bus Selector1 : BusSelector  OutputSignals=psir
  Gain : Gain  Gain=car.cts
  Minus : Sum  Inputs=+-
  cts : Outport
  wires:
  psi_f/1 -> Bus Selector/1
  psi_r/1 -> Bus Selector1/1
  Bus Selector/1 -> Minus/1  "<psif>"
  Bus Selector1/1 -> Minus/2  "<psir>"
  Minus/1 -> Gain/1
  Gain/1 -> cts/1  "cts"

== system dynamic/Roll, Pitch, Heave/Ground ==
  Bus Creator1 : BusCreator  Inputs=8
  Constant{,1..7} (8 alike) : Constant  Value=0
  Z0 : Outport
  wires:
  Constant1/1 -> Bus Creator1/2  "Z0_fr"
  Constant2/1 -> Bus Creator1/3  "Z0_rl"
  Constant4/1 -> Bus Creator1/5  "Z0dot_fl"
  Constant5/1 -> Bus Creator1/6  "Z0dot_fr"
  Constant7/1 -> Bus Creator1/8  "Z0dot_rr"
  Constant/1 -> Bus Creator1/1  "Z0_fl"
  Bus Creator1/1 -> Z0/1  "Z0"
  Constant6/1 -> Bus Creator1/7  "Z0dot_rl"
  Constant3/1 -> Bus Creator1/4  "Z0_rr"

== system dynamic/Roll, Pitch, Heave/Heave ==
  Zf : Inport
  Bus Creator : BusCreator  Inputs=3
  Bus Selector : BusSelector  OutputSignals=Zf_fl,Zf_fr,Zf_rl,Zf_rr
  Constant : Constant  Value=car.g
  Gain : Gain  Gain=car.ms
  Gain1 : Gain  Gain=1/car.ms
  Integrator : Integrator  InitialCondition=Zsdot0
  Integrator1 : Integrator  InitialCondition=Zs0
  Minus : Sum  Inputs=++++-
  Heave : Outport
  wires:
  Minus/1 -> Gain1/1
  Integrator1/1 -> Bus Creator/1  "Zscg"
  Bus Creator/1 -> Heave/1  "Zscg"
  Integrator/1 -> Integrator1/1, Bus Creator/2  "Zscgdot"
  Zf/1 -> Bus Selector/1
  Bus Selector/1 -> Minus/1  "<Zf_fl>"
  Bus Selector/2 -> Minus/2  "<Zf_fr>"
  Bus Selector/3 -> Minus/3  "<Zf_rl>"
  Bus Selector/4 -> Minus/4  "<Zf_rr>"
  Constant/1 -> Gain/1
  Gain/1 -> Minus/5
  Gain1/1 -> Integrator/1, Bus Creator/3  "Zscgddot"

== system dynamic/Roll, Pitch, Heave/Pitch moment ==
  FX : Inport
  Bus Selector : BusSelector  OutputSignals=FXfl_b,FXfr_b,FXrr_b,FXrl_b
  Gain : Gain  Gain=-car.cgh
  Minus : Sum  Inputs=++++
  Pitch moment : Outport
  wires:
  Gain/1 -> Pitch moment/1  "M_pitch"
  FX/1 -> Bus Selector/1
  Bus Selector/1 -> Minus/1  "<FXfl_b>"
  Bus Selector/2 -> Minus/2  "<FXfr_b>"
  Bus Selector/3 -> Minus/3  "<FXrr_b>"
  Bus Selector/4 -> Minus/4  "<FXrl_b>"
  Minus/1 -> Gain/1

== system dynamic/Roll, Pitch, Heave/Roll front ==
  Zf : Inport
  M_roll : Inport  Port=2
  M_cts : Inport  Port=3
  Bus Creator : BusCreator  Inputs=3
  Bus Selector : BusSelector  OutputSignals=Zf_fl,Zf_fr
  Bus Selector1 : BusSelector  OutputSignals=M_roll_f
  Gain : Gain  Gain=car.r.fr
  Gain1 : Gain  Gain=car.r.fl
  Gain2 : Gain  Gain=car.Ixxf
  Integrator : Integrator  InitialCondition=psifdot0
  Integrator1 : Integrator  InitialCondition=psif0
  Minus : Sum  Inputs=+-+-
  psi front : Outport
  wires:
  Integrator/1 -> Bus Creator/2, Integrator1/1  "psifdot"
  Bus Creator/1 -> psi front/1  "psif"
  Integrator1/1 -> Bus Creator/1  "psif"
  Minus/1 -> Gain2/1
  Zf/1 -> Bus Selector/1
  Bus Selector/2 -> Gain/1  "<Zf_fr>"
  Gain/1 -> Minus/2
  Bus Selector/1 -> Gain1/1  "<Zf_fl>"
  Gain1/1 -> Minus/1
  M_cts/1 -> Minus/4
  Gain2/1 -> Bus Creator/3, Integrator/1  "psifddot"
  M_roll/1 -> Bus Selector1/1
  Bus Selector1/1 -> Minus/3  "<M_roll_f>"

== system dynamic/Roll, Pitch, Heave/Roll moment ==
  FY : Inport
  Bus Creator : BusCreator  Inputs=4
  Bus Selector : BusSelector  OutputSignals=FYfr_b,FYfl_b,FYrr_b,FYrl_b
  Constant : Constant  Value=car.cgh
  Constant1 : Constant  Value=car.rch.f
  Constant2 : Constant  Value=car.cgh
  Constant3 : Constant  Value=car.rch.r
  Gain : Gain  Gain=car.rch.f
  Gain1 : Gain  Gain=car.rch.r
  Minus : Sum  Inputs=+-
  Minus1 : Sum  Inputs=+-
  Minus2 : Sum
  Minus3 : Sum
  Product : Product
  Product1 : Product
  Roll moment : Outport
  wires:
  Minus/1 -> Product/2
  Gain/1 -> Bus Creator/3  "M_inelas_f"
  Product/1 -> Bus Creator/1  "M_roll_f"
  Constant/1 -> Minus/1
  Constant3/1 -> Minus1/2
  Constant1/1 -> Minus/2
  Product1/1 -> Bus Creator/2  "M_roll_r"
  Minus1/1 -> Product1/2
  Constant2/1 -> Minus1/1
  Gain1/1 -> Bus Creator/4  "M_inelas_r"
  Bus Creator/1 -> Roll moment/1  "Roll moment"
  FY/1 -> Bus Selector/1
  Bus Selector/1 -> Minus2/1  "<FYfr_b>"
  Bus Selector/2 -> Minus2/2  "<FYfl_b>"
  Minus2/1 -> Gain/1, Product/1
  Bus Selector/3 -> Minus3/1  "<FYrr_b>"
  Bus Selector/4 -> Minus3/2  "<FYrl_b>"
  Minus3/1 -> Gain1/1, Product1/1

== system dynamic/Roll, Pitch, Heave/Roll rear ==
  Zf : Inport
  M_roll : Inport  Port=2
  M_cts : Inport  Port=3
  Bus Creator : BusCreator  Inputs=3
  Bus Selector : BusSelector  OutputSignals=Zf_rl,Zf_rr
  Bus Selector1 : BusSelector  OutputSignals=M_roll_r
  Gain : Gain  Gain=car.r.fr
  Gain1 : Gain  Gain=car.r.fl
  Gain2 : Gain  Gain=1/car.Ixxr
  Integrator : Integrator  InitialCondition=psirdot0
  Integrator1 : Integrator  InitialCondition=psir0
  Minus : Sum  Inputs=+-++
  psi rear : Outport
  wires:
  Minus/1 -> Gain2/1
  Integrator1/1 -> Bus Creator/1  "psir"
  Bus Creator/1 -> psi rear/1  "psir"
  Integrator/1 -> Integrator1/1, Bus Creator/2  "psirdot"
  Bus Selector1/1 -> Minus/3  "<M_roll_r>"
  Bus Selector/2 -> Gain/1  "<Zf_rr>"
  Gain1/1 -> Minus/1
  M_roll/1 -> Bus Selector1/1
  Bus Selector/1 -> Gain1/1  "<Zf_rl>"
  Gain/1 -> Minus/2
  Zf/1 -> Bus Selector/1
  M_cts/1 -> Minus/4
  Gain2/1 -> Integrator/1, Bus Creator/3  "psirddot"

== system dynamic/Roll, Pitch, Heave/Unsprung ==
  Zf : Inport
  Z0 : Inport  Port=2
  Bus Creator : BusCreator  Inputs=4
  Bus Creator1 : BusCreator  Inputs=4
  Unsprung fl : Subsystem
  Unsprung flr : Subsystem
  Unsprung rl : Subsystem
  Unsprung rr : Subsystem
  Zu : Outport
  FZ : Outport  Port=2
  wires:
  Z0/1 -> Unsprung flr/2(Z0), Unsprung rr/2(Z0), Unsprung rl/2(Z0), Unsprung fl/2(Z0)
  Zf/1 -> Unsprung rr/1(Zf), Unsprung rl/1(Zf), Unsprung flr/1(Zf), Unsprung fl/1(Zf)
  Unsprung fl/1(Zu_fl) -> Bus Creator/1
  Unsprung flr/1(Zu_fr) -> Bus Creator/2
  Unsprung rl/1(Zu_rl) -> Bus Creator/3
  Unsprung rr/1(Zu_rr) -> Bus Creator/4
  Bus Creator/1 -> Zu/1  "Zu"
  Unsprung fl/2(FZ_fl) -> Bus Creator1/1
  Unsprung flr/2(FZ_fr) -> Bus Creator1/2
  Unsprung rl/2(FZ_rl) -> Bus Creator1/3
  Unsprung rr/2(FZ_rr) -> Bus Creator1/4
  Bus Creator1/1 -> FZ/1  "FZ"

== system dynamic/Roll, Pitch, Heave/Zs ==
  Zscg : Inport
  psi_f : Inport  Port=2
  psi_r : Inport  Port=3
  rho : Inport  Port=4
  Bus Creator : BusCreator  Inputs=8
  Bus Selector : BusSelector  OutputSignals=Zscg,Zscgdot
  Bus Selector1 : BusSelector  OutputSignals=psif,psifdot
  Bus Selector2 : BusSelector  OutputSignals=psir,psirdot
  Bus Selector3 : BusSelector  OutputSignals=rho,rhodot
  Subsystem1 : Subsystem
  Subsystem4 : Subsystem
  Zs : Outport
  wires:
  Bus Creator/1 -> Zs/1  "Zs"
  Subsystem4/1(Zs_fl) -> Bus Creator/1
  Subsystem4/2(Zs_fr) -> Bus Creator/2
  Subsystem4/3(Zs_rl) -> Bus Creator/3
  Subsystem4/4(Zs_rr) -> Bus Creator/4
  Zscg/1 -> Bus Selector/1
  Bus Selector/1 -> Subsystem4/1(Zscg)  "<Zscg>"
  psi_f/1 -> Bus Selector1/1
  Bus Selector1/1 -> Subsystem4/2(psi_f)  "<psif>"
  psi_r/1 -> Bus Selector2/1
  Bus Selector2/1 -> Subsystem4/3(psi_r)  "<psir>"
  rho/1 -> Bus Selector3/1
  Bus Selector3/1 -> Subsystem4/4(rho)  "<rho>"
  Bus Selector/2 -> Subsystem1/1(Zscgdot)  "<Zscgdot>"
  Bus Selector1/2 -> Subsystem1/2(psi_fdot)  "<psifdot>"
  Bus Selector2/2 -> Subsystem1/3(psi_rdot)  "<psirdot>"
  Bus Selector3/2 -> Subsystem1/4(rhodot)  "<rhodot>"
  Subsystem1/1(Zsdot_fl) -> Bus Creator/5
  Subsystem1/2(Zsdot_fr) -> Bus Creator/6
  Subsystem1/3(Zsdot_rl) -> Bus Creator/7
  Subsystem1/4(Zsdot_rr) -> Bus Creator/8

== system dynamic/Roll, Pitch, Heave/corner forces ==
  Zs : Inport
  Zu : Inport  Port=2
  M_roll : Inport  Port=3
  M_arb : Inport  Port=4
  Bus Creator : BusCreator  Inputs=4
  Zs_fl : Subsystem
  Zs_fr : Subsystem
  Zs_rl : Subsystem
  Zs_rr : Subsystem
  Zf : Outport
  wires:
  Zs_rl/1(Zf_rl) -> Bus Creator/3
  Zs_fr/1(Zf_fr) -> Bus Creator/2
  M_roll/1 -> Zs_fl/3(M_roll), Zs_fr/1(M_roll), Zs_rl/1(M_roll), Zs_rr/1(M_roll)
  Zs_rr/1(Zf_rr) -> Bus Creator/4
  Zs_fl/1(Zf_fl) -> Bus Creator/1
  Bus Creator/1 -> Zf/1  "Zf"
  M_arb/1 -> Zs_rl/2(M_arb), Zs_fr/2(M_arb), Zs_fl/4(M_arb), Zs_rr/2(M_arb)
  Zs/1 -> Zs_rr/3(Zs), Zs_rl/3(Zs), Zs_fr/3(Zs), Zs_fl/1(Zs)
  Zu/1 -> Zs_rr/4(Zu), Zs_rl/4(Zu), Zs_fr/4(Zu), Zs_fl/2(Zu)

== system dynamic/Roll, Pitch, Heave/pitch ==
  Zf : Inport
  M_pitch : Inport  Port=2
  Bus Creator : BusCreator  Inputs=3
  Bus Selector : BusSelector  OutputSignals=Zf_fl,Zf_fr,Zf_rl,Zf_rr
  Gain : Gain  Gain=1/car.Iyy
  Gain1 : Gain  Gain=car.a
  Gain2 : Gain  Gain=car.b
  Integrator : Integrator  InitialCondition=rhodot0
  Integrator1 : Integrator  InitialCondition=rho0
  Minus : Sum  Inputs=-++
  Minus1 : Sum
  Minus2 : Sum
  rho : Outport
  wires:
  Integrator/1 -> Bus Creator/2, Integrator1/1  "rhodot"
  Bus Creator/1 -> rho/1  "rho"
  Integrator1/1 -> Bus Creator/1  "rho"
  Gain/1 -> Bus Creator/3, Integrator/1  "rhoddot"
  Minus/1 -> Gain/1
  Zf/1 -> Bus Selector/1
  Bus Selector/1 -> Minus1/1  "<Zf_fl>"
  Bus Selector/2 -> Minus1/2  "<Zf_fr>"
  Bus Selector/3 -> Minus2/1  "<Zf_rl>"
  Bus Selector/4 -> Minus2/2  "<Zf_rr>"
  Minus1/1 -> Gain1/1
  Gain1/1 -> Minus/1
  Minus2/1 -> Gain2/1
  Gain2/1 -> Minus/2
  M_pitch/1 -> Minus/3

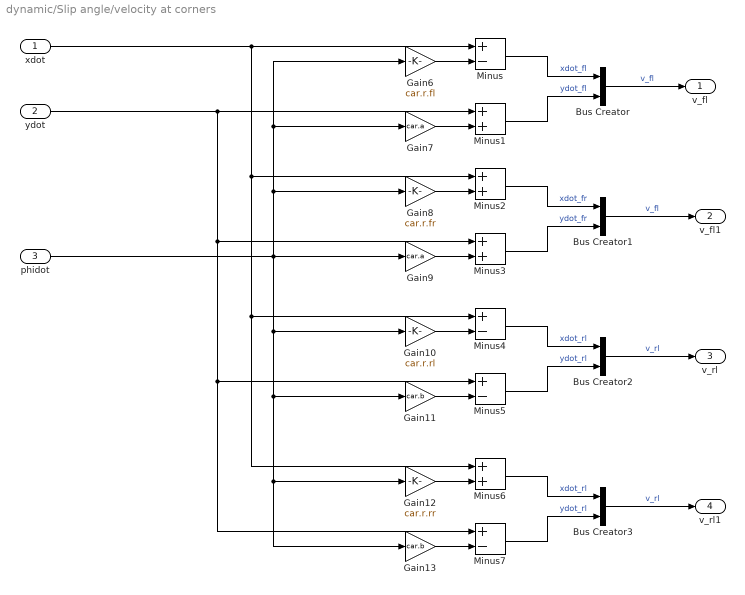
== system dynamic/Slip angle/velocity at corners ==
  xdot : Inport
  ydot : Inport  Port=2
  phidot : Inport  Port=3
  Bus Creator{,1..3} (4 alike) : BusCreator  Inputs=2
  Gain10 : Gain  Gain=car.r.rl
  Gain11 : Gain  Gain=car.b
  Gain12 : Gain  Gain=car.r.rr
  Gain13 : Gain  Gain=car.b
  Gain6 : Gain  Gain=car.r.fl
  Gain7 : Gain  Gain=car.a
  Gain8 : Gain  Gain=car.r.fr
  Gain9 : Gain  Gain=car.a
  Minus{,4..5,7} (4 alike) : Sum  Inputs=+-
  Minus{1..3,6} (4 alike) : Sum
  v_fl : Outport
  v_fl1 : Outport  Port=2
  v_rl : Outport  Port=3
  v_rl1 : Outport  Port=4
  wires:
  ydot/1 -> Minus7/1, Minus5/1, Minus3/1, Minus1/1
  Gain8/1 -> Minus2/2
  Gain7/1 -> Minus1/2
  phidot/1 -> Gain7/1, Gain6/1, Gain8/1, Gain13/1, Gain12/1, Gain11/1, Gain10/1, Gain9/1
  Minus2/1 -> Bus Creator1/1  "xdot_fr"
  xdot/1 -> Minus6/1, Minus4/1, Minus2/1, Minus/1
  Minus1/1 -> Bus Creator/2  "ydot_fl"
  Gain9/1 -> Minus3/2
  Gain10/1 -> Minus4/2
  Gain11/1 -> Minus5/2
  Minus5/1 -> Bus Creator2/2  "ydot_rl"
  Minus4/1 -> Bus Creator2/1  "xdot_rl"
  Gain12/1 -> Minus6/2
  Minus7/1 -> Bus Creator3/2  "ydot_rl"
  Minus6/1 -> Bus Creator3/1  "xdot_rl"
  Gain13/1 -> Minus7/2
  Minus/1 -> Bus Creator/1  "xdot_fl"
  Gain6/1 -> Minus/2
  Minus3/1 -> Bus Creator1/2  "ydot_fr"
  Bus Creator2/1 -> v_rl/1  "v_rl"
  Bus Creator3/1 -> v_rl1/1  "v_rl"
  Bus Creator1/1 -> v_fl1/1  "v_fl"
  Bus Creator/1 -> v_fl/1  "v_fl"

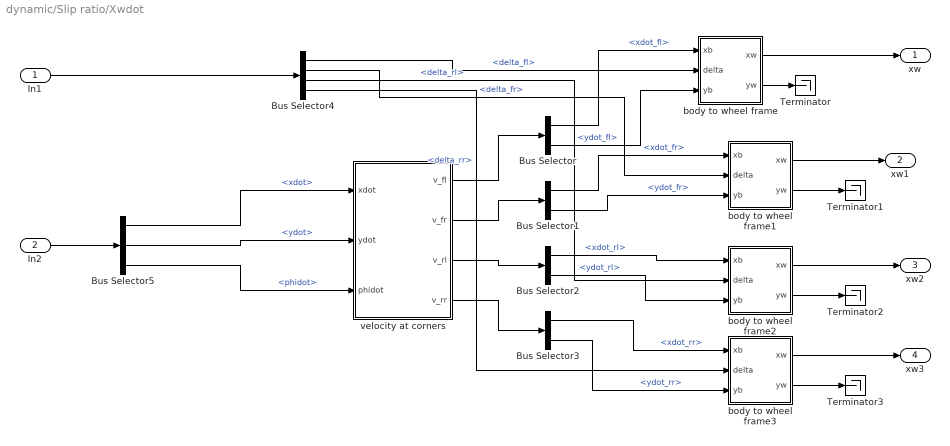
== system dynamic/Slip ratio/Xwdot ==
  In1 : Inport
  In2 : Inport  Port=2
  Bus Selector : BusSelector  OutputSignals=xdot_fl,ydot_fl
  Bus Selector1 : BusSelector  OutputSignals=xdot_fr,ydot_fr
  Bus Selector2 : BusSelector  OutputSignals=xdot_rl,ydot_rl
  Bus Selector3 : BusSelector  OutputSignals=xdot_rr,ydot_rr
  Bus Selector4 : BusSelector  OutputSignals=delta_fl,delta_fr,delta_rl,delta_rr
  Bus Selector5 : BusSelector  OutputSignals=xdot,ydot,phidot
  Terminator{,1..3} (4 alike) : Terminator
  body to wheel frame : Subsystem
  body to wheel frame1 : Subsystem
  body to wheel frame2 : Subsystem
  body to wheel frame3 : Subsystem
  velocity at corners : Subsystem
  xw : Outport
  xw1 : Outport  Port=2
  xw2 : Outport  Port=3
  xw3 : Outport  Port=4
  wires:
  body to wheel frame/2(yw) -> Terminator/1
  velocity at corners/1(v_fl) -> Bus Selector/1
  velocity at corners/3(v_rl) -> Bus Selector2/1
  Bus Selector/2 -> body to wheel frame/3(yb)  "<ydot_fl>"
  velocity at corners/2(v_fr) -> Bus Selector1/1
  Bus Selector5/3 -> velocity at corners/3(phidot)  "<phidot>"
  Bus Selector3/2 -> body to wheel frame3/3(yb)  "<ydot_rr>"
  body to wheel frame1/2(yw) -> Terminator1/1
  Bus Selector4/1 -> body to wheel frame/2(delta)  "<delta_fl>"
  velocity at corners/4(v_rr) -> Bus Selector3/1
  body to wheel frame2/1(xw) -> xw2/1
  Bus Selector/1 -> body to wheel frame/1(xb)  "<xdot_fl>"
  body to wheel frame/1(xw) -> xw/1
  body to wheel frame3/2(yw) -> Terminator3/1
  Bus Selector2/1 -> body to wheel frame2/1(xb)  "<xdot_rl>"
  Bus Selector5/2 -> velocity at corners/2(ydot)  "<ydot>"
  Bus Selector3/1 -> body to wheel frame3/1(xb)  "<xdot_rr>"
  Bus Selector5/1 -> velocity at corners/1(xdot)  "<xdot>"
  Bus Selector4/2 -> body to wheel frame1/2(delta)  "<delta_fr>"
  In1/1 -> Bus Selector4/1
  body to wheel frame2/2(yw) -> Terminator2/1
  Bus Selector4/3 -> body to wheel frame2/2(delta)  "<delta_rl>"
  Bus Selector2/2 -> body to wheel frame2/3(yb)  "<ydot_rl>"
  Bus Selector4/4 -> body to wheel frame3/2(delta)  "<delta_rr>"
  Bus Selector1/1 -> body to wheel frame1/1(xb)  "<xdot_fr>"
  In2/1 -> Bus Selector5/1
  Bus Selector1/2 -> body to wheel frame1/3(yb)  "<ydot_fr>"
  body to wheel frame1/1(xw) -> xw1/1
  body to wheel frame3/1(xw) -> xw3/1

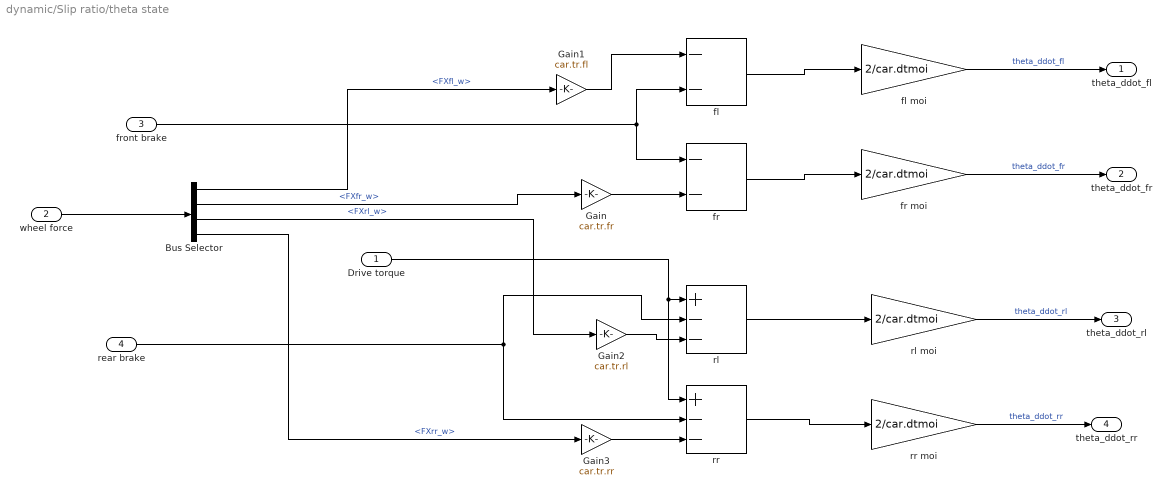
== system dynamic/Slip ratio/theta state ==
  Drive torque : Inport
  wheel force : Inport  Port=2
  front brake : Inport  Port=3
  rear brake : Inport  Port=4
  Bus Selector : BusSelector  OutputSignals=FXfl_w,FXfr_w,FXrl_w,FXrr_w
  Gain : Gain  Gain=car.tr.fr
  Gain1 : Gain  Gain=car.tr.fl
  Gain2 : Gain  Gain=car.tr.rl
  Gain3 : Gain  Gain=car.tr.rr
  fl : Sum  Inputs=--
  fl moi : Gain  Gain=2/car.dtmoi
  fr : Sum  Inputs=--
  fr moi : Gain  Gain=2/car.dtmoi
  rl : Sum  Inputs=+--
  rl moi : Gain  Gain=2/car.dtmoi
  rr : Sum  Inputs=+--
  rr moi : Gain  Gain=2/car.dtmoi
  theta_ddot_fl : Outport
  theta_ddot_fr : Outport  Port=2
  theta_ddot_rl : Outport  Port=3
  theta_ddot_rr : Outport  Port=4
  wires:
  fr/1 -> fr moi/1
  rl/1 -> rl moi/1
  rr/1 -> rr moi/1
  rear brake/1 -> rr/2, rl/2
  fl/1 -> fl moi/1
  front brake/1 -> fl/2, fr/1
  fl moi/1 -> theta_ddot_fl/1  "theta_ddot_fl"
  fr moi/1 -> theta_ddot_fr/1  "theta_ddot_fr"
  rl moi/1 -> theta_ddot_rl/1  "theta_ddot_rl"
  rr moi/1 -> theta_ddot_rr/1  "theta_ddot_rr"
  wheel force/1 -> Bus Selector/1
  Bus Selector/1 -> Gain1/1  "<FXfl_w>"
  Bus Selector/2 -> Gain/1  "<FXfr_w>"
  Bus Selector/3 -> Gain2/1  "<FXrl_w>"
  Bus Selector/4 -> Gain3/1  "<FXrr_w>"
  Gain1/1 -> fl/1
  Gain/1 -> fr/2
  Gain2/1 -> rl/3
  Gain3/1 -> rr/3
  Drive torque/1 -> rr/1, rl/1

== system dynamic/Vehicle model/wheel to body frame fl ==
  xw : Inport
  delta : Inport  Port=2
  yw : Inport  Port=3
  Cos : Trigonometry  Operator=cos
  Cos1 : Trigonometry
  Gain : Gain  Gain=pi/180
  Minus : Sum  Inputs=+-
  Minus1 : Sum
  Product{,1..3} (4 alike) : Product
  xb : Outport
  yb : Outport  Port=2
  wires:
  Minus1/1 -> yb/1
  xw/1 -> Product/1, Product2/1
  Product/1 -> Minus/1
  Product3/1 -> Minus1/2
  Minus/1 -> xb/1
  delta/1 -> Gain/1
  Product1/1 -> Minus/2
  yw/1 -> Product1/2, Product3/1
  Cos1/1 -> Product1/1, Product2/2
  Product2/1 -> Minus1/1
  Cos/1 -> Product/2, Product3/2
  Gain/1 -> Cos/1, Cos1/1

== system dynamic/Vehicle model/wheel to body frame fr ==
  xw : Inport
  delta : Inport  Port=2
  yw : Inport  Port=3
  Cos : Trigonometry  Operator=cos
  Cos1 : Trigonometry
  Gain : Gain  Gain=pi/180
  Minus : Sum  Inputs=+-
  Minus1 : Sum
  Product{,1..3} (4 alike) : Product
  xb : Outport
  yb : Outport  Port=2
  wires:
  Cos/1 -> Product3/2, Product/2
  Product2/1 -> Minus1/1
  Cos1/1 -> Product2/2, Product1/1
  yw/1 -> Product3/1, Product1/2
  Product1/1 -> Minus/2
  delta/1 -> Gain/1
  Minus/1 -> xb/1
  Product3/1 -> Minus1/2
  Product/1 -> Minus/1
  xw/1 -> Product2/1, Product/1
  Minus1/1 -> yb/1
  Gain/1 -> Cos1/1, Cos/1

== system dynamic/Vehicle model/wheel to body frame rl ==
  xw : Inport
  delta : Inport  Port=2
  yw : Inport  Port=3
  Cos : Trigonometry  Operator=cos
  Cos1 : Trigonometry
  Gain : Gain  Gain=pi/180
  Minus : Sum  Inputs=+-
  Minus1 : Sum
  Product{,1..3} (4 alike) : Product
  xb : Outport
  yb : Outport  Port=2
  wires:
  Minus1/1 -> yb/1
  xw/1 -> Product/1, Product2/1
  Product/1 -> Minus/1
  Product3/1 -> Minus1/2
  Minus/1 -> xb/1
  delta/1 -> Gain/1
  Product1/1 -> Minus/2
  yw/1 -> Product1/2, Product3/1
  Cos1/1 -> Product1/1, Product2/2
  Product2/1 -> Minus1/1
  Cos/1 -> Product/2, Product3/2
  Gain/1 -> Cos/1, Cos1/1

== system dynamic/Vehicle model/wheel to body frame rr ==
  xw : Inport
  delta : Inport  Port=2
  yw : Inport  Port=3
  Cos : Trigonometry  Operator=cos
  Cos1 : Trigonometry
  Gain : Gain  Gain=pi/180
  Minus : Sum  Inputs=+-
  Minus1 : Sum
  Product{,1..3} (4 alike) : Product
  xb : Outport
  yb : Outport  Port=2
  wires:
  Cos/1 -> Product3/2, Product/2
  Product2/1 -> Minus1/1
  Cos1/1 -> Product2/2, Product1/1
  yw/1 -> Product3/1, Product1/2
  Product1/1 -> Minus/2
  delta/1 -> Gain/1
  Minus/1 -> xb/1
  Product3/1 -> Minus1/2
  Product/1 -> Minus/1
  xw/1 -> Product2/1, Product/1
  Minus1/1 -> yb/1
  Gain/1 -> Cos1/1, Cos/1

== system dynamic/Roll, Pitch, Heave/Unsprung/Unsprung fl ==
  Zf : Inport
  Z0 : Inport  Port=2
  Bus Creator : BusCreator  Inputs=3
  Bus Selector : BusSelector  OutputSignals=Zf_fl
  Bus Selector1 : BusSelector  OutputSignals=Z0_fl,Z0dot_fl
  Constant : Constant  Value=car.g
  Gain : Gain  Gain=car.K.t
  Gain1 : Gain  Gain=car.c.t
  Gain2 : Gain  Gain=1/car.mufl
  Gain4 : Gain  Gain=car.mufl
  Integrator : Integrator  InitialCondition=Zufldot0
  Integrator1 : Integrator  InitialCondition=Zufl0
  Minus : Sum  Inputs=----
  Minus1 : Sum  Inputs=+-
  Minus2 : Sum  Inputs=+-
  Minus3 : Sum
  Zu_fl : Outport
  FZ_fl : Outport  Port=2
  wires:
  Z0/1 -> Bus Selector1/1
  Zf/1 -> Bus Selector/1
  Bus Selector/1 -> Minus/1  "<Zf_fl>"
  Bus Selector1/1 -> Minus1/2  "<Z0_fl>"
  Minus1/1 -> Gain/1
  Gain/1 -> Minus3/1, Minus/2
  Bus Selector1/2 -> Minus2/2  "<Z0dot_fl>"
  Minus2/1 -> Gain1/1
  Gain1/1 -> Minus3/2, Minus/3
  Minus/1 -> Gain2/1
  Gain2/1 -> Bus Creator/3, Integrator/1  "Zufl_ddot"
  Integrator/1 -> Minus2/1, Bus Creator/2, Integrator1/1  "Zufl_dot"
  Integrator1/1 -> Minus1/1, Bus Creator/1  "Zufl"
  Bus Creator/1 -> Zu_fl/1  "Zu_fl"
  Gain4/1 -> Minus/4
  Constant/1 -> Gain4/1
  Minus3/1 -> FZ_fl/1  "FZ_fl"

== system dynamic/Roll, Pitch, Heave/Unsprung/Unsprung flr ==
  Zf : Inport
  Z0 : Inport  Port=2
  Bus Creator : BusCreator  Inputs=3
  Bus Selector : BusSelector  OutputSignals=Zf_fr
  Bus Selector1 : BusSelector  OutputSignals=Z0_fr,Z0dot_fr
  Constant : Constant  Value=car.g
  Gain : Gain  Gain=car.K.t
  Gain1 : Gain  Gain=car.c.t
  Gain2 : Gain  Gain=1/car.mufr
  Gain4 : Gain  Gain=car.mufr
  Integrator : Integrator  InitialCondition=Zufrdot0
  Integrator1 : Integrator  InitialCondition=Zufr0
  Minus : Sum  Inputs=----
  Minus1 : Sum  Inputs=+-
  Minus2 : Sum  Inputs=+-
  Minus3 : Sum
  Zu_fr : Outport
  FZ_fr : Outport  Port=2
  wires:
  Constant/1 -> Gain4/1
  Gain4/1 -> Minus/4
  Bus Creator/1 -> Zu_fr/1  "Zu_fr"
  Integrator1/1 -> Bus Creator/1, Minus1/1  "Zufr"
  Integrator/1 -> Integrator1/1, Bus Creator/2, Minus2/1  "Zufr_dot"
  Gain2/1 -> Integrator/1, Bus Creator/3  "Zufr_ddot"
  Minus/1 -> Gain2/1
  Gain1/1 -> Minus/3, Minus3/2
  Minus2/1 -> Gain1/1
  Bus Selector1/2 -> Minus2/2  "<Z0dot_fr>"
  Gain/1 -> Minus3/1, Minus/2
  Minus1/1 -> Gain/1
  Bus Selector1/1 -> Minus1/2  "<Z0_fr>"
  Bus Selector/1 -> Minus/1  "<Zf_fr>"
  Zf/1 -> Bus Selector/1
  Z0/1 -> Bus Selector1/1
  Minus3/1 -> FZ_fr/1  "FZ_fr"
